simulink model "PEMcell"  (R2024b)
settings: Solver=VariableStepAuto  StartTime=0.0  StopTime=10  RelTol=1e-3
settings Model: Creator=hp  LastModifiedBy=hp
settings SolverCC: AlgebraicLoopSolver=TrustRegion
settings DebuggingCC: UnconnectedInputMsg=warning  UnconnectedOutputMsg=warning  UnconnectedLineMsg=warning
settings ModelReferenceCC: EnableRefExpFcnMdlSchedulingChecks=on
settings RTWCC: GPUComputeCapability=3.5  DLArmComputeVersion=19.05

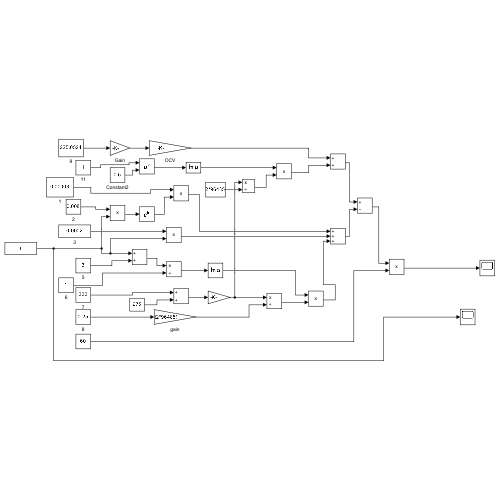
[thumbnail: Simulink's stored preview of the top-level diagram]
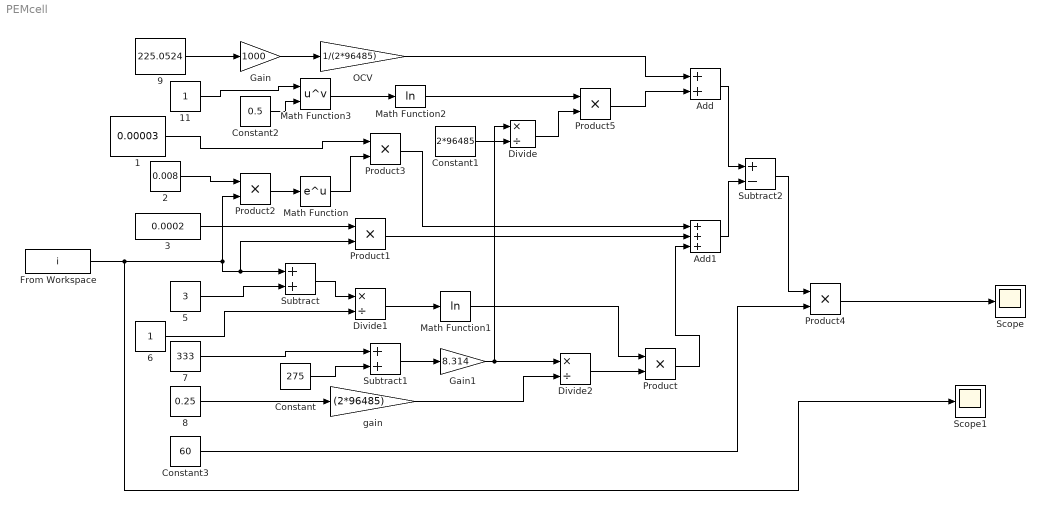
== system PEMcell ==
  1 : Constant  Value=0.00003
  11 : Constant
  2 : Constant  Value=0.008
  3 : Constant  Value=0.0002
  5 : Constant  Value=3
  6 : Constant
  7 : Constant  Value=333
  8 : Constant  Value=0.25
  9 : Constant  Value=225.0524
  Add : Sum
  Add1 : Sum  Inputs=+++
  Constant : Constant  Value=275
  Constant1 : Constant  Value=2*96485
  Constant2 : Constant  Value=0.5
  Constant3 : Constant  Value=60
  Divide : Product  Inputs=*/
  Divide1 : Product  Inputs=*/
  Divide2 : Product  Inputs=*/
  From Workspace : FromWorkspace  VariableName=i
  Gain : Gain  Gain=1000
  Gain1 : Gain  Gain=8.314
  Math Function : Math  SignedPower=on  RndMeth=Zero
  Math Function1 : Math  Operator=log
  Math Function2 : Math  Operator=log
  Math Function3 : Math  Operator=pow
  OCV : Gain  Gain=1/(2*96485)
  Product{,1..5} (6 alike) : Product
  Scope : Scope
  Scope1 : Scope
  Subtract : Sum
  Subtract1 : Sum
  Subtract2 : Sum  Inputs=+-
  gain : Gain  Gain=(2*96485)
  wires:
  Gain/1 -> OCV/1
  OCV/1 -> Add/1
  Product5/1 -> Add/2
  9/1 -> Gain/1
  11/1 -> Math Function3/1
  Constant2/1 -> Math Function3/2
  Math Function3/1 -> Math Function2/1
  Math Function2/1 -> Product5/1
  Divide/1 -> Product5/2
  Constant1/1 -> Divide/2
  1/1 -> Product3/1
  2/1 -> Product2/1
  Product2/1 -> Math Function/1
  Math Function/1 -> Product3/2
  3/1 -> Product1/1
  5/1 -> Subtract/2
  Product1/1 -> Add1/2
  6/1 -> Divide1/2
  Subtract/1 -> Divide1/1
  Divide1/1 -> Math Function1/1
  Constant/1 -> Subtract1/2
  Subtract1/1 -> Gain1/1
  Gain1/1 -> Divide/1, Divide2/1
  Product3/1 -> Add1/1
  Divide2/1 -> Product/2
  Product/1 -> Add1/3
  Add1/1 -> Subtract2/2
  Add/1 -> Subtract2/1
  8/1 -> gain/1
  gain/1 -> Divide2/2
  Math Function1/1 -> Product/1
  7/1 -> Subtract1/1
  Constant3/1 -> Product4/2
  Subtract2/1 -> Product4/1
  Product4/1 -> Scope/1
  From Workspace/1 -> Scope1/1, Product2/2, Product1/2, Subtract/1
